simulink model "LTS_testing"  (R2025b)
settings: Solver=ode23t  StartTime=0.0  StopTime=1
model workspace: external: MATLAB File C:\Users\thoma\Documents\ME-Steering-2026\MATLAB\VD\LTS.m (data not in the file)
undefined symbols (not defined in the file): AR26
libraries: vehdynlibtire x4, autolibshared x2, vehdynlibdriver x1, simulink x1, autolibmappedmotor x1, autolibsharedcoupling x1, vehdynlibsteering x1
(part 1 of 2)
settings Model: Creator=thoma  LastModifiedBy=thoma
settings SolverCC: ZeroCrossControl=DisableAll
settings DebuggingCC: UnderSpecifiedDimensionMsg=warning

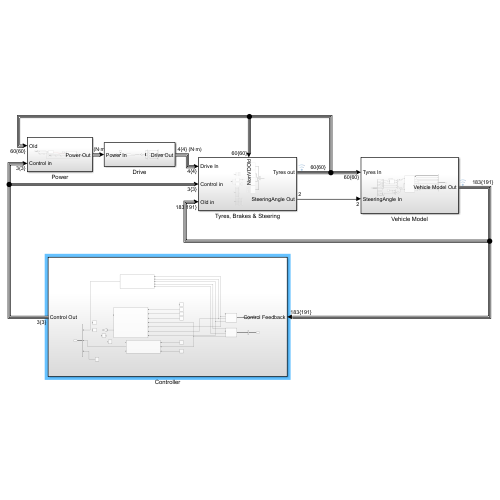
[thumbnail: Simulink's stored preview of the top-level diagram]
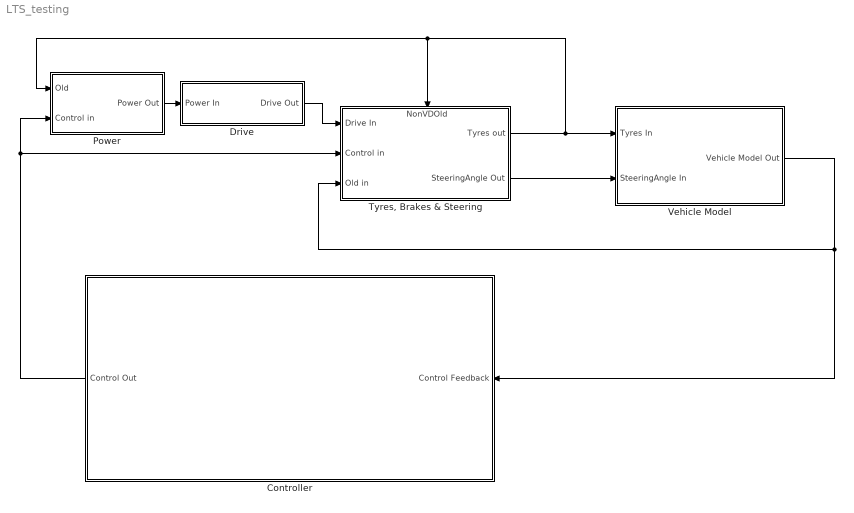
== system LTS_testing ==
  Controller : Subsystem
  Drive : Subsystem
  Power : Subsystem
  "Tyres, Brakes & Steering" : Subsystem
      settings: PortSchema="{\"entries\":[{\"content\":{\"sides\":[{\"content\":{\"connectorIds\":[\"In1\",\"In2\",\"In3\"]},\"type\":\"ConnectorPlacement.EquallySpacedRectSide\",\"uuid\":\"2d0cea8b-83c5-43d0-a9da-df7959890b84\"},{\"content\":{\"connectorIds\":[\"Out1\",\"Out2\"],\"side\":\"RIGHT\"},\"type\":\"ConnectorPlacement.EquallySpacedRectSide\",\"uuid\":\"18a5ce0c-4f74-4e1c-9a31-f96c275e466d\"},{\"content\":{\"connectorIds\":[\"In4\"],\"side\":\"TOP\"},\"type\":\"ConnectorPlacement.EquallySpacedRectSide\",\"uuid\":\"ac68a692-bd3e-4c2d-9cd0-6d8aee15298d\"}]},\"type\":\"ConnectorPlacement.EquallySpacedConnector\",\"uuid\":\"5a266ba3-3c83-4752-af97-895e1d69d679\"}],\"packageUris\":[\"http://schema.mathworks.com/mf0/Connector/R2020b\"],\"version\":\"1.0\"}"
  Vehicle Model : Subsystem
  wires:
  Controller/1(Control Out) -> Power/2(Control in), "Tyres, Brakes & Steering"/2(Control in)
  Drive/1(Drive Out) -> "Tyres, Brakes & Steering"/1(Drive In)
  Power/1(Power Out) -> Drive/1(Power In)
  "Tyres, Brakes & Steering"/1(Tyres out) -> Power/1(Old), "Tyres, Brakes & Steering"/4(NonVDOld), Vehicle Model/1(Tyres In)
  Vehicle Model/1(Vehicle Model Out) -> Controller/1(Control Feedback), "Tyres, Brakes & Steering"/3(Old in)
  "Tyres, Brakes & Steering"/2(SteeringAngle Out) -> Vehicle Model/2(SteeringAngle In)

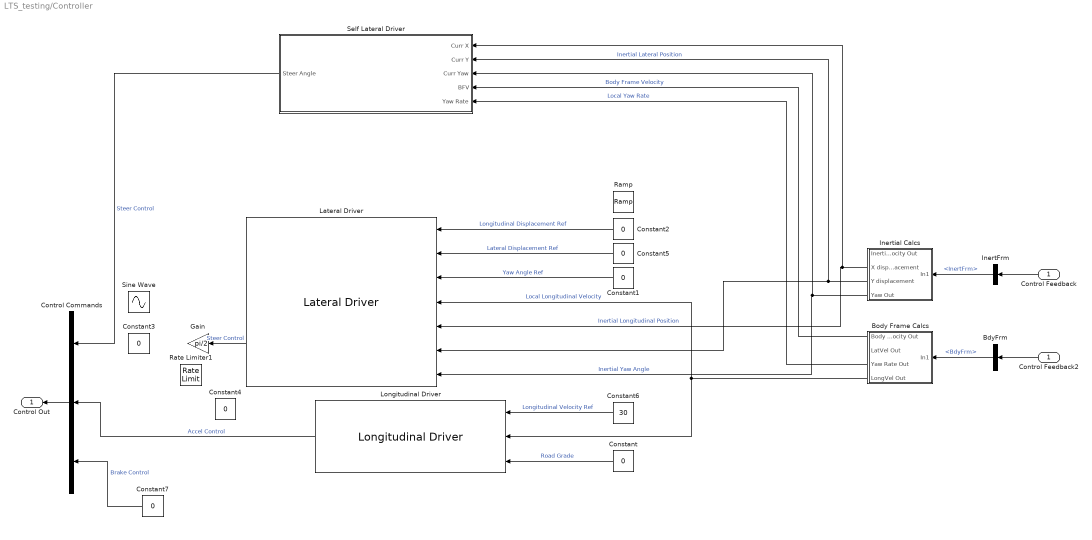
== system LTS_testing/Controller ==
  Control Feedback : Inport
  BdyFrm : BusSelector  OutputSignals=Info.BdyFrm
  Body Frame Calcs : Subsystem
  Constant{,1..5,7} (7 alike) : Constant  Value=0
  Constant6 : Constant  Value=30
  Control Commands : BusCreator  Inputs=3
  Control Feedback2 : InportShadow
  Gain : Gain  Gain=pi/2
  InertFrm : BusSelector  OutputSignals=Info.InertFrm
  Inertial Calcs : Subsystem
  Lateral Driver : vehdynlibdriver/Lateral Driver  extSteerOvr=off  extSteerHld=off  extSteerZero=off  steerOut=off  cntrlTypeLat=Stanley  coordMode=SAE J670 (Z-down)  angUnits=rad  tau=0.1  L=3  vecPose=off  dynamMode=off  PositionGainF=2.5  PositionGainR=2.5  YawRateGain=.2  DelayGain=.2  a=AR26.aLength  b=AR26.bLength  m=AR26.Mass  Cy_f=35000  Cy_r=40000  I=120  Ksteer=18  theta=30*pi/180  aMode=2
  Longitudinal Driver : autolibshared/Longitudinal Driver  extAccelOvr=off  extDecelOvr=off  extAccelHld=off  extDecelHld=off  extAccelZero=off  extDecelZero=off  cntrlType=PI  shftType=None  velUnits=m/s  gearOut=off  Kp=0.7  Ki=0.05  Kff=.1  Kg=0  VehVelVec=[0 100]  KffVec=[.1 .1]  KpVec=[10 10]  KiVec=[5 5]  KgVec=[0 0]  m=1500  Kpt=3000  tau=.1  L=2  aR=200  bR=2.5  cR=.5  g=9.81  vnom=5  Kaw=1  tauerr=.01  tauPt=2  GearInit=0  tShift=.1  pdlVec=[0.1 0.4 0.5 0.9]  upShftTbl=[-1 12.9375 26.4375 39.9375 51.18749999999999 62.4375 72.84375 83.25;-1 16.3125 29.8125 43.3125 54.5624 65.8125 76.78125 87.75;-1 19.6875 33.1875 46.68749999999999 57.9375 69.1875 80.71875 92.25;-1 33 52.5 77.25 100.5 138.75 161.875 185]  dwnShftTbl=[1 9.5625 23.0625 36.5625 47.8125 59.0625 68.90625 78.75;1 12.9375 26.4375 39.9375 51.18749999999999 62.4375 72.84375 83.25;1 16.3125 29.8125 43.3125 54.562499 65.8125 76.78125 87.75;1 19.6875 33.1875 46.68749999999999 57.9375 69.1875 80.71875 92.25]  tClutch=.5  tRev=.5  tPark=120  aMode=2  UpGearVec="[0  1  2  3  4  5  6  7]"  DownGearVec="[1  2  3  4  5  6  7  8]"
      settings: LibrarySourceBlock=vehdynlibdriver/Longitudinal Driver
  Ramp : simulink/Sources/Ramp  slope=35  start=15  InitialOutput=0
  Rate Limiter1 : RateLimiter  RisingSlewLimit=0.5  SampleTimeMode=inherited
  Self Lateral Driver : Subsystem
  Sine Wave : Sin  Amplitude=1.6  Frequency=0.5  SampleTime=0
  Control Out : Outport
  wires:
  Control Commands/1 -> Control Out/1
  Control Feedback/1 -> InertFrm/1
  Control Feedback2/1 -> BdyFrm/1
  Constant/1 -> Longitudinal Driver/3  "Road Grade"
  Constant6/1 -> Longitudinal Driver/1  "Longitudinal Velocity Ref"
  Longitudinal Driver/2 -> Control Commands/2  "Accel Control"
  Constant7/1 -> Control Commands/3  "Brake Control"
  BdyFrm/1 -> Body Frame Calcs/1(In1)  "<BdyFrm>"
  Constant5/1 -> Lateral Driver/2  "Lateral Displacement Ref"
  InertFrm/1 -> Inertial Calcs/1(In1)  "<InertFrm>"
  Inertial Calcs/3(Y displacement) -> Self Lateral Driver/2(Curr Y), Lateral Driver/6  "Inertial Lateral Position"
  Inertial Calcs/4(Yaw Out) -> Self Lateral Driver/3(Curr Yaw), Lateral Driver/7  "Inertial Yaw Angle"
  Body Frame Calcs/4(LongVel Out) -> Longitudinal Driver/2, Lateral Driver/4  "Local Longitudinal Velocity"
  Constant1/1 -> Lateral Driver/3  "Yaw Angle Ref"
  Constant2/1 -> Lateral Driver/1  "Longitudinal Displacement Ref"
  Inertial Calcs/2(X displacement) -> Self Lateral Driver/1(Curr X), Lateral Driver/5  "Inertial Longitudinal Position"
  Lateral Driver/2 -> Gain/1  "Steer Control"
  Body Frame Calcs/1(Body Frame Velocity Out) -> Self Lateral Driver/4(BFV)  "Body Frame Velocity"
  Self Lateral Driver/1(Steer Angle) -> Control Commands/1  "Steer Control"
  Body Frame Calcs/3(Yaw Rate Out) -> Self Lateral Driver/5(Yaw Rate)  "Local Yaw Rate"

== system LTS_testing/Drive ==
  Power In : Inport
  Bus Creator : BusCreator  Inputs=4
  Bus Selector : BusSelector  OutputSignals=Motor Torque (Nm)
  Display : Display
  Gain : Gain
  Gear Ratio : Gain  Gain=AR26.GearRatio
  Multiply{1..4} (4 alike) : Gain
  Drive Out : Outport
  wires:
  Power In/1 -> Bus Selector/1
  Bus Selector/1 -> Gear Ratio/1, Display/1  "<Motor Torque (Nm)>"
  Gear Ratio/1 -> Gain/1
  Multiply4/1 -> Bus Creator/1  "FLDriveTrq"
  Multiply3/1 -> Bus Creator/4  "RRDriveTrq"
  Multiply1/1 -> Bus Creator/2  "FRDriveTrq"
  Multiply2/1 -> Bus Creator/3  "RLDriveTrq"
  Bus Creator/1 -> Drive Out/1
  Gain/1 -> Multiply4/1, Multiply1/1, Multiply3/1, Multiply2/1

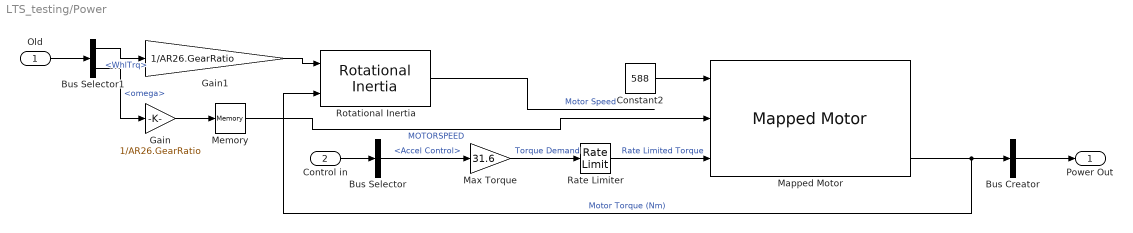
== system LTS_testing/Power ==
  Old : Inport
  Control in : Inport  Port=2
  Bus Creator : BusCreator  Inputs=1
  Bus Selector : BusSelector  OutputSignals=Accel Control
  Bus Selector1 : BusSelector  OutputSignals=FL_Dyn.WhlTrq,FL_Dyn.omega
  Constant2 : Constant  Value=588
  Gain : Gain  Gain=1/AR26.GearRatio
  Gain1 : Gain  Gain=1/AR26.GearRatio
  Mapped Motor : autolibmappedmotor/Mapped Motor  w_Tmax_bp_ext=w_Tmax_bp  Tmax_w_V_ext=Tmax_w_V  w_Tmin_bp_ext=w_Tmin_bp  Tmin_w_V_ext=Tmin_w_V  port_config=Speed  param_by=Maximum torque and power  w_t=[ 0 375 750 800 ]  T_t=[0.09 0.08 0.07 0]  torque_max=31.6  power_max=20000  SpreadsheetTqLimitsFileName=MotorCalibrationImportData.xlsx  Tmax_w_V=[0.09 0.09 0.09;0.08 0.08 0.08;0.07 0.07 0.07;0 0 0]  w_Tmax_bp=[ 0 375 750 800 ]  V_Tmax_bp=[500 750 900]  Tmin_w_V=[-0.09 -0.09 -0.09;-0.08 -0.08 -0.08;-0.07 -0.07 -0.07;0 0 0]  w_Tmin_bp=[ 0 375 750 800 ]  V_Tmin_bp=[500 750 900]  Tc=0.02  param_loss=Single efficiency measurement  SpreadsheetLossFileName=MotorCalibrationImportData.xlsx  SpreadsheetEffFileName=MotorCalibrationImportData.xlsx  eff=95  w_eff=375  T_eff=0.08  Piron=0  Pbase=0  w_eff_bp=[-8000 -4000 0 4000 8000]  T_eff_bp=[0 0.03 0.06 0.09]  Temp_eff_bp=[233.15 293.15 373.15]  V_eff_bp=[500 700 900]  losses_table=[1.49 1.67 2.21 3.10; 0.42 0.69 1.14 2.03; 0.06 0.24 0.78 1.68; 0.42 0.69 1.14 2.03; 1.49 1.67 2.21 3.10]  losses_table_3d=cat(3,1.05*[1.49 1.67 2.21 3.10; 0.42 0.69 1.14 2.03; 0.06 0.24 0.78 1.68; 0.42 0.69 1.14 2.03; 1.49 1.67 2.21 3.10],[1.49 1.67 2.21 3.10; 0.42 0.69 1.14 2.03; 0.06 0.24 0.78 1.68; 0.42 0.69 1.14 2.03; 1.49 1.67 2.21 3.10],1.03*[1.49 1.67 2.21 3.10; 0.42 0.69 1.14 2.03; 0.06 0.24 0.78 1.68; 0.42 0.69 1.14 2.03; 1.49 1.67 2.21 3.10])  losses_table_4d=cat(4,cat(3,[1.5645 0.441 0.063 0.441 1.5645;1.7535 0.7245 0.252 0.7245 1.7535;2.3205 1.197 0.819 1.197 2.3205;3.255 2.1315 1.764 2.1315 3.255],[1.5645 0.441 0.063 0.441 1.5645;1.7535 0.7245 0.252 0.7245 1.7535;2.3205 1.197 0.819 1.197 2.3205;3.255 2.1315 1.764 2.1315 3.255],[1.5645 0.441 0.063 0.441 1.5645;1.7535 0.7245 0.252 0.7245 1.7535;2.3205 1.197 0.819 1.197 2.3205;3.255 2.1315 1.764 2.1315 3.255]),cat(3,[1.49 0.42 0.06 0.42 1.49;1.67 0.69 0.24 0.69 1.67;2.21 1.14 0.78 1.14 2.21;3.1 2.03 1.68 2.03 3.1],[1.49 0.42 0.06 0.42 1.49;1.67 0.69 0.24 0.69 1.67;2.21 1.14 0.78 1.14 2.21;3.1 2.03 1.68 2.03 3.1],[1.49 0.42 0.06 0.42 1.49;1.67 0.69 0.24 0.69 1.67;2.21 1.14 0.78 1.14 2.21;3.1 2.03 1.68 2.03 3.1]),cat(3,[1.5347 0.4326 0.0618 0.4326 1.5347;1.7201 0.7107 0.2472 0.7107 1.7201;2.2763 1.1742 0.8034 1.1742 2.2763;3.193 2.0909 1.7304 2.0909 3.193],[1.5347 0.4326 0.0618 0.4326 1.5347;1.7201 0.7107 0.2472 0.7107 1.7201;2.2763 1.1742 0.8034 1.1742 2.2763;3.193 2.0909 1.7304 2.0909 3.193],[1.5347 0.4326 0.0618 0.4326 1.5347;1.7201 0.7107 0.2472 0.7107 1.7201;2.2763 1.1742 0.8034 1.1742 2.2763;3.193 2.0909 1.7304 2.0909 3.193]))  efficiency_table=[95 95 95 95; 95 95 95 95; 95 95 95 95; 95 95 95 95; 95 95 95 95]  efficiency_table_3d=cat(3,90*ones(5,4),95*ones(5,4),92*ones(5,4))  efficiency_table_4d=cat(4,cat(3,90*ones(5,4)',90*ones(5,4)',90*ones(5,4)'),cat(3,95*ones(5,4)',95*ones(5,4)',95*ones(5,4)'),cat(3,92*ones(5,4)',92*ones(5,4)',92*ones(5,4)'))  J=5e-6  b=1e-5  omega_o=0  T_t_extended=[0 0.07 0.08 0.09 0.08 0.07 0]  w_t_extended=[-800 -750 -375 0 375 750 800]  KLossIron=0  KLossCopper=0  x_w_eff_vec=[-8000 -4000 0 4000 8000]  x_T_eff_vec=[-0.09 -0.06 -0.03 0 0.03 0.06 0.09]  x_tmp_eff_vec=[233.15 293.15 373.15]  x_V_eff_vec=[500 700 900]  x_losses_mat=[3.1 2.21 1.67 1.49 1.67 2.21 3.1;2.03 1.14 0.69 0.42 0.69 1.14 2.03;1.68 0.78 0.24 0.06 0.24 0.78 1.68;2.03 1.14 0.69 0.42 0.69 1.14 2.03;3.1 2.21 1.67 1.49 1.67 2.21 3.1]  x_losses_mat_3d=cat(3,[3.255 2.3205 1.7535 1.5645 1.7535 2.3205 3.255;2.1315 1.197 0.7245 0.441 0.7245 1.197 2.1315;1.764 0.819 0.252 0.063 0.252 0.819 1.764;2.1315 1.197 0.7245 0.441 0.7245 1.197 2.1315;3.255 2.3205 1.7535 1.5645 1.7535 2.3205 3.255],[3.1 2.21 1.67 1.49 1.67 2.21 3.1;2.03 1.14 0.69 0.42 0.69 1.14 2.03;1.68 0.78 0.24 0.06 0.24 0.78 1.68;2.03 1.14 0.69 0.42 0.69 1.14 2.03;3.1 2.21 1.67 1.49 1.67 2.21 3.1],[3.193 2.2763 1.7201 1.5347 1.7201 2.2763 3.193;2.0909 1.1742 0.7107 0.4326 0.7107 1.1742 2.0909;1.7304 0.8034 0.2472 0.0618 0.2472 0.8034 1.7304;2.0909 1.1742 0.7107 0.4326 0.7107 1.1742 2.0909;3.193 2.2763 1.7201 1.5347 1.7201 2.2763 3.193])  x_losses_mat_4d=cat(4,cat(3,[1.5645 0.441 0.063 0.441 1.5645;1.7535 0.7245 0.252 0.7245 1.7535;2.3205 1.197 0.819 1.197 2.3205;3.255 2.1315 1.764 2.1315 3.255],[1.5645 0.441 0.063 0.441 1.5645;1.7535 0.7245 0.252 0.7245 1.7535;2.3205 1.197 0.819 1.197 2.3205;3.255 2.1315 1.764 2.1315 3.255],[1.5645 0.441 0.063 0.441 1.5645;1.7535 0.7245 0.252 0.7245 1.7535;2.3205 1.197 0.819 1.197 2.3205;3.255 2.1315 1.764 2.1315 3.255]),cat(3,[1.49 0.42 0.06 0.42 1.49;1.67 0.69 0.24 0.69 1.67;2.21 1.14 0.78 1.14 2.21;3.1 2.03 1.68 2.03 3.1],[1.49 0.42 0.06 0.42 1.49;1.67 0.69 0.24 0.69 1.67;2.21 1.14 0.78 1.14 2.21;3.1 2.03 1.68 2.03 3.1],[1.49 0.42 0.06 0.42 1.49;1.67 0.69 0.24 0.69 1.67;2.21 1.14 0.78 1.14 2.21;3.1 2.03 1.68 2.03 3.1]),cat(3,[1.5347 0.4326 0.0618 0.4326 1.5347;1.7201 0.7107 0.2472 0.7107 1.7201;2.2763 1.1742 0.8034 1.1742 2.2763;3.193 2.0909 1.7304 2.0909 3.193],[1.5347 0.4326 0.0618 0.4326 1.5347;1.7201 0.7107 0.2472 0.7107 1.7201;2.2763 1.1742 0.8034 1.1742 2.2763;3.193 2.0909 1.7304 2.0909 3.193],[1.5347 0.4326 0.0618 0.4326 1.5347;1.7201 0.7107 0.2472 0.7107 1.7201;2.2763 1.1742 0.8034 1.1742 2.2763;3.193 2.0909 1.7304 2.0909 3.193]))  CalLossMapData={}  CalLossWithTempMapData={}  aMode=2  RefBlkName='autolibmappedmotor/Mapped Motor'
      settings: LibrarySourceBlock=vdynlib/Powertrain/Propulsion/Mapped Motor
  Max Torque : Gain  Gain=31.6
  Memory : Memory
  Rate Limiter : RateLimiter  RisingSlewLimit=0.1  FallingSlewLimit=-100  SampleTimeMode=inherited
  Rotational Inertia : autolibsharedcoupling/Rotational Inertia  port_config=Simulink  extInfo=off  externJ=off  J=.01  b=.001  omega_o=0  blkID=0  aMode=2
      settings: LibrarySourceBlock=vdynlib/Powertrain/Drivetrain/Couplings/Rotational Inertia
  Power Out : Outport
  wires:
  Constant2/1 -> Mapped Motor/1
  Old/1 -> Bus Selector1/1
  Mapped Motor/3 -> Rotational Inertia/2, Bus Creator/1  "Motor Torque (Nm)"
  Bus Creator/1 -> Power Out/1
  Control in/1 -> Bus Selector/1
  Bus Selector/1 -> Max Torque/1  "<Accel Control>"
  Max Torque/1 -> Rate Limiter/1  "Torque Demand"
  Rotational Inertia/1 -> ?  "Motor Speed"
  Bus Selector1/1 -> Gain1/1  "<WhlTrq>"
  Gain1/1 -> Rotational Inertia/1
  Rate Limiter/1 -> Mapped Motor/3  "Rate Limited Torque"
  Bus Selector1/2 -> Gain/1  "<omega>"
  Gain/1 -> Memory/1
  Memory/1 -> Mapped Motor/2  "MOTORSPEED"

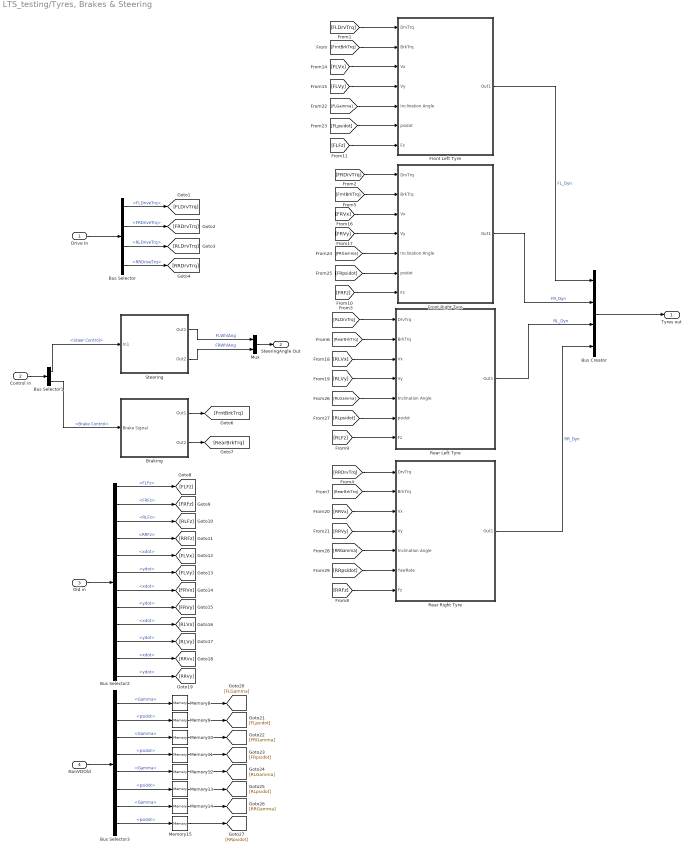
== system LTS_testing/Tyres, Brakes & Steering ==
  Drive In : Inport
  Control in : Inport  Port=2
  Old in : Inport  Port=3
  NonVDOld : Inport  Port=4
  Braking : Subsystem
  Bus Creator : BusCreator  Inputs=4
  Bus Selector : BusSelector  OutputSignals=FLDriveTrq,FRDriveTrq,RLDriveTrq,RRDriveTrq
  Bus Selector1 : BusSelector  OutputSignals=Steer Control,Brake Control
  Bus Selector2 : BusSelector  OutputSignals=FLFz,FRFz,RLFz,RRFz,Info.BdyFrm.FrntAxl.Lft.Vel.xdot,Info.BdyFrm.FrntAxl.Lft.Vel.ydot,Info.BdyFrm.FrntAxl.Rght.Vel.xdot,Info.BdyFrm.FrntAxl.Rght.Vel.ydot,Info.BdyFrm.RearAxl.Lft.Vel.xdot,Info.BdyFrm.RearAxl.Lft.Vel.ydot,Info.BdyFrm.RearAxl.Rght.Vel.xdot,Info.BdyFrm.RearAxl.Rght.Vel.ydot
  Bus Selector3 : BusSelector  OutputSignals=FL_Dyn.Gamma,FL_Dyn.psidot,FR_Dyn.Gamma,FR_Dyn.psidot,RL_Dyn.Gamma,RL_Dyn.psidot,RR_Dyn.Gamma,RR_Dyn.psidot
  Front Left Tyre : Subsystem
  Front Right Tyre : Subsystem
  Memory{8..15} (8 alike) : Memory
  Mux : Mux  Inputs=2
  Rear Left Tyre : Subsystem
  Rear Right Tyre : Subsystem
  Steering : Subsystem
  Tyres out : Outport
  SteeringAngle Out : Outport  Port=2
  wires:
  Bus Creator/1 -> Tyres out/1
  Front Left Tyre/1(Out1) -> Bus Creator/1  "FL_Dyn"
  Front Right Tyre/1(Out1) -> Bus Creator/2  "FR_Dyn"
  Rear Left Tyre/1(Out1) -> Bus Creator/3  "RL_Dyn"
  Rear Right Tyre/1(Out1) -> Bus Creator/4  "RR_Dyn"
  Control in/1 -> Bus Selector1/1
  Bus Selector1/1 -> Steering/1(In1)  "<Steer Control>"
  Steering/1(Out1) -> Mux/1  "FLWhlAng"
  Steering/2(Out2) -> Mux/2  "FRWhlAng"
  Braking/1(Out1) -> [FrntBrkTrq]
  Braking/2(Out2) -> [RearBrkTrq]
  Bus Selector/1 -> [FLDrvTrq]  "<FLDriveTrq>"
  Drive In/1 -> Bus Selector/1
  Bus Selector/4 -> [RRDrvTrq]  "<RRDriveTrq>"
  Bus Selector/3 -> [RLDrvTrq]  "<RLDriveTrq>"
  Bus Selector/2 -> [FRDrvTrq]  "<FRDriveTrq>"
  [FLDrvTrq] -> Front Left Tyre/1(DrvTrq)
  [FrntBrkTrq] -> Front Left Tyre/2(BrkTrq)
  [FRDrvTrq] -> Front Right Tyre/1(DrvTrq)
  [FrntBrkTrq] -> Front Right Tyre/2(BrkTrq)
  [RLDrvTrq] -> Rear Left Tyre/1(DrvTrq)
  [RearBrkTrq] -> Rear Left Tyre/2(BrkTrq)
  [RRDrvTrq] -> Rear Right Tyre/1(DrvTrq)
  [RearBrkTrq] -> Rear Right Tyre/2(BrkTrq)
  Bus Selector1/2 -> Braking/1(Brake Signal)  "<Brake Control>"
  [FRFz] -> Front Right Tyre/7(Fz)
  [RLFz] -> Rear Left Tyre/7(Fz)
  [RRFz] -> Rear Right Tyre/7(Fz)
  Old in/1 -> Bus Selector2/1
  [FLFz] -> Front Left Tyre/7(Fz)
  [FRGamma] -> Front Right Tyre/5(Inclination Angle)
  [FLGamma] -> Front Left Tyre/5(Inclination Angle)
  [RLGamma] -> Rear Left Tyre/5(Inclination Angle)
  [RRGamma] -> Rear Right Tyre/5(Inclination Angle)
  [RLVx] -> Rear Left Tyre/3(Vx)
  [RLVy] -> Rear Left Tyre/4(Vy)
  [RRVx] -> Rear Right Tyre/3(Vx)
  [RRVy] -> Rear Right Tyre/4(Vy)
  [FLVy] -> Front Left Tyre/4(Vy)
  [FLVx] -> Front Left Tyre/3(Vx)
  [FRVy] -> Front Right Tyre/4(Vy)
  [FRVx] -> Front Right Tyre/3(Vx)
  NonVDOld/1 -> Bus Selector3/1
  Bus Selector3/1 -> Memory8/1  "<Gamma>"
  Bus Selector3/2 -> Memory9/1  "<psidot>"
  Bus Selector3/3 -> Memory10/1  "<Gamma>"
  Bus Selector3/4 -> Memory11/1  "<psidot>"
  Bus Selector3/5 -> Memory12/1  "<Gamma>"
  Bus Selector3/6 -> Memory13/1  "<psidot>"
  Bus Selector3/7 -> Memory14/1  "<Gamma>"
  Bus Selector3/8 -> Memory15/1  "<psidot>"
  Memory8/1 -> [FLGamma]
  Memory9/1 -> [FLpsidot]
  [FLpsidot] -> Front Left Tyre/6(psidot)
  [FRpsidot] -> Front Right Tyre/6(psidot)
  [RLpsidot] -> Rear Left Tyre/6(psidot)
  [RRpsidot] -> Rear Right Tyre/6(YawRate)
  Memory10/1 -> [FRGamma]
  Memory11/1 -> [FRpsidot]
  Memory12/1 -> [RLGamma]
  Memory13/1 -> [RLpsidot]
  Memory14/1 -> [RRGamma]
  Memory15/1 -> [RRpsidot]
  Bus Selector2/2 -> [FRFz]  "<FRFz>"
  Bus Selector2/3 -> [RLFz]  "<RLFz>"
  Bus Selector2/5 -> [FLVx]  "<xdot>"
  Bus Selector2/6 -> [FLVy]  "<ydot>"
  Bus Selector2/7 -> [FRVx]  "<xdot>"
  Bus Selector2/8 -> [FRVy]  "<ydot>"
  Bus Selector2/9 -> [RLVx]  "<xdot>"
  Bus Selector2/10 -> [RLVy]  "<ydot>"
  Bus Selector2/11 -> [RRVx]  "<xdot>"
  Bus Selector2/12 -> [RRVy]  "<ydot>"
  Bus Selector2/1 -> [FLFz]  "<FLFz>"
  Bus Selector2/4 -> [RRFz]  "<RRFz>"
  Mux/1 -> SteeringAngle Out/1

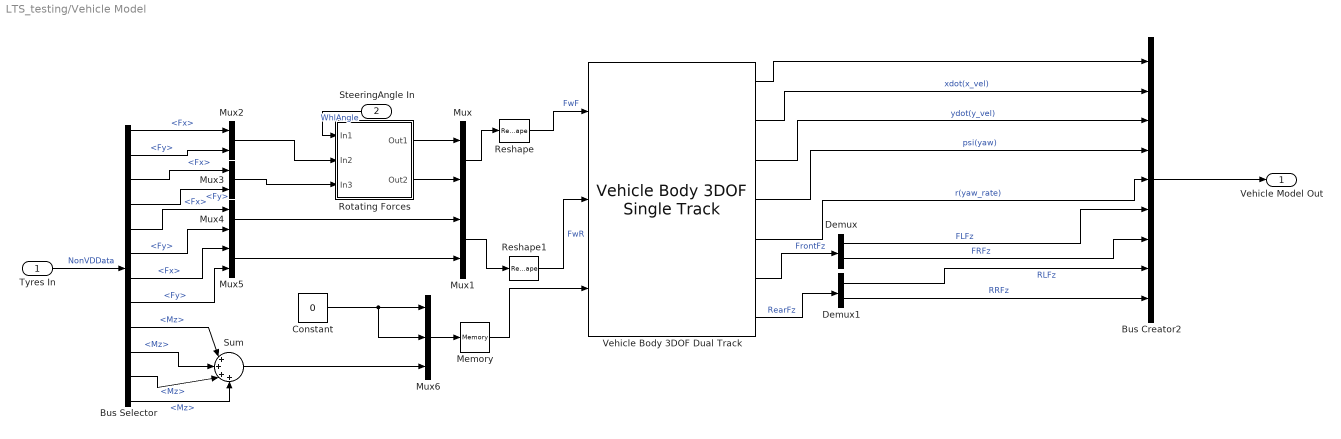
== system LTS_testing/Vehicle Model ==
  Tyres In : Inport
  SteeringAngle In : Inport  Port=2
  Bus Creator2 : BusCreator  Inputs=9
  Bus Selector : BusSelector  OutputSignals=FL_Dyn.Fx,FL_Dyn.Fy,FR_Dyn.Fx,FR_Dyn.Fy,RL_Dyn.Fx,RL_Dyn.Fy,RR_Dyn.Fx,RR_Dyn.Fy,FL_Dyn.Mz,FR_Dyn.Mz,RL_Dyn.Mz,RR_Dyn.Mz
  Constant : Constant  Value=0
  Demux : Demux  Outputs=2
  Demux1 : Demux  Outputs=2
  Memory : Memory
  Mux{,1..5} (6 alike) : Mux  Inputs=2
  Mux6 : Mux  Inputs=3
  Reshape : Reshape  OutputDimensionality=Customize  OutputDimensions=[2,2]
  Reshape1 : Reshape  OutputDimensionality=Customize  OutputDimensions=[2,2]
  Rotating Forces : Subsystem
  Sum : Sum  Inputs=|++++
  Vehicle Body 3DOF Dual Track : autolibshared/Vehicle Body 3DOF Single Track  trackMode=Dual  inputMode=External forces  frontSteerMode=off  rearSteerMode=off  windMode=off  muMode=off  extFMode=off  extMMode=on  htchFMode=off  htchMMode=off  extXo=off  extpsio=off  extxdoto=off  extro=off  extYo=off  extTamb=off  extydoto=off  aMode=2  NF=2  NR=2  m=AR26.Mass  a=AR26.aLength  b=AR26.bLength  h=AR26.CGHeight  dh=1  hh=0.2  X_o=0  xdot_o=AR26.Vx0  CalphaMode=off  sigmaMode=on  d=AR26.CGLateral  hl=0  w=[AR26.FrontTrackwidth,AR26.RearTrackWidth]  Cy_f=12e3  Cy_r=11e3  sigma_f=.1  sigma_r=.1  alpha_f_brk=[-0.785, -0.628, -0.471, -0.314, -0.157, 0.000, 0.157, 0.314, 0.471, 0.628, 0.785]  Cy_f_data=[2000, 3000, 4000, 5500, 7000, 9000, 7000, 5500, 4000, 3000, 2000]  alpha_r_brk=[-0.785, -0.628, -0.471, -0.314, -0.157, 0.000, 0.157, 0.314, 0.471, 0.628, 0.785]  Cy_r_data=[2000, 3000, 4000, 5500, 7000, 9000, 7000, 5500, 4000, 3000, 2000]  Y_o=0  ydot_o=0  Izz=AR26.Izz  psi_o=0  r_o=0  Af=0.81  Cd=1.4  Cl=4.230  Cpm=.1  beta_w=[0 0.01:0.01:0.3]  Cs=[0:0.03:0.9]  Cym=[0 1e-6:0.01:0.3]  Pabs=101325  Tair=273  g=9.81  mu=1  xdot_tol=.01  Fznom=5000  Fxtire_sat=7e4  Fytire_sat=7e4  longOff=0  latOff=0  vertOff=0  wrapAng=off
      settings: LibrarySourceBlock=vehdynlibeom/Vehicle Body 3DOF Dual Track
  Vehicle Model Out : Outport
  wires:
  Tyres In/1 -> Bus Selector/1  "NonVDData"
  Bus Selector/3 -> Mux3/1  "<Fx>"
  Bus Selector/5 -> Mux4/1  "<Fx>"
  Bus Selector/7 -> Mux5/1  "<Fx>"
  Vehicle Body 3DOF Dual Track/2 -> Bus Creator2/2  "xdot(x_vel)"
  Vehicle Body 3DOF Dual Track/7 -> Demux1/1  "RearFz"
  Vehicle Body 3DOF Dual Track/3 -> Bus Creator2/3  "ydot(y_vel)"
  Vehicle Body 3DOF Dual Track/4 -> Bus Creator2/4  "psi(yaw)"
  Vehicle Body 3DOF Dual Track/5 -> Bus Creator2/5  "r(yaw_rate)"
  Vehicle Body 3DOF Dual Track/6 -> Demux/1  "FrontFz"
  Demux/1 -> Bus Creator2/6  "FLFz"
  Demux/2 -> Bus Creator2/7  "FRFz"
  Demux1/1 -> Bus Creator2/8  "RLFz"
  Demux1/2 -> Bus Creator2/9  "RRFz"
  Bus Selector/1 -> Mux2/1  "<Fx>"
  Bus Selector/2 -> Mux2/2  "<Fy>"
  Bus Selector/4 -> Mux3/2  "<Fy>"
  Bus Selector/6 -> Mux4/2  "<Fy>"
  Bus Selector/8 -> Mux5/2  "<Fy>"
  Mux/1 -> Reshape/1
  Mux1/1 -> Reshape1/1
  Bus Creator2/1 -> Vehicle Model Out/1
  Vehicle Body 3DOF Dual Track/1 -> Bus Creator2/1
  Mux2/1 -> Rotating Forces/2(In2)
  Mux3/1 -> Rotating Forces/3(In3)
  Mux4/1 -> Mux1/1
  Mux5/1 -> Mux1/2
  SteeringAngle In/1 -> Rotating Forces/1(In1)  "WhlAngle"
  Reshape1/1 -> Vehicle Body 3DOF Dual Track/2  "FwR"
  Reshape/1 -> Vehicle Body 3DOF Dual Track/1  "FwF"
  Rotating Forces/1(Out1) -> Mux/1
  Rotating Forces/2(Out2) -> Mux/2
  Bus Selector/9 -> Sum/1  "<Mz>"
  Bus Selector/10 -> Sum/2  "<Mz>"
  Bus Selector/11 -> Sum/3  "<Mz>"
  Bus Selector/12 -> Sum/4  "<Mz>"
  Sum/1 -> Mux6/3
  Constant/1 -> Mux6/2, Mux6/1
  Mux6/1 -> Memory/1
  Memory/1 -> Vehicle Body 3DOF Dual Track/3

== system LTS_testing/Controller/Body Frame Calcs ==
  In1 : Inport
  Bus Selector : BusSelector  OutputSignals=Cg.Vel.xdot,Cg.Vel.ydot,FrntAxl.Steer.WhlAngFL,FrntAxl.Steer.WhlAngFR,Cg.Ang.Beta,Cg.AngVel.r,Cg.DCM
  Integrator : Integrator
  Integrator1 : Integrator
  Velocity : Math  Operator=hypot
  Body Frame Velocity Out : Outport
  LatVel Out : Outport  Port=2
  Yaw Rate Out : Outport  Port=3
  LongVel Out : Outport  Port=4
  wires:
  In1/1 -> Bus Selector/1
  Bus Selector/2 -> Velocity/2, Integrator1/1, LatVel Out/1  "<ydot>"
  Bus Selector/1 -> LongVel Out/1, Integrator/1, Velocity/1  "<xdot>"
  Velocity/1 -> Body Frame Velocity Out/1  "Body Frame Velocity"
  Bus Selector/6 -> Yaw Rate Out/1  "<r>"

== system LTS_testing/Controller/Inertial Calcs ==
  In1 : Inport
  Bus Selector : BusSelector  OutputSignals=Cg.Vel.Xdot,Cg.Vel.Ydot,Cg.Ang.psi,Cg.Disp.X,Cg.Disp.Y
  Hypot : Math  Operator=hypot
  Inertial Velocity Out : Outport
  X displacement : Outport  Port=2
  Y displacement : Outport  Port=3
  Yaw Out : Outport  Port=4
  wires:
  In1/1 -> Bus Selector/1
  Bus Selector/2 -> Hypot/2  "<Ydot>"
  Bus Selector/1 -> Hypot/1  "<Xdot>"
  Hypot/1 -> Inertial Velocity Out/1
  Bus Selector/3 -> Yaw Out/1  "<psi>"
  Bus Selector/4 -> X displacement/1  "<X>"
  Bus Selector/5 -> Y displacement/1  "<Y>"

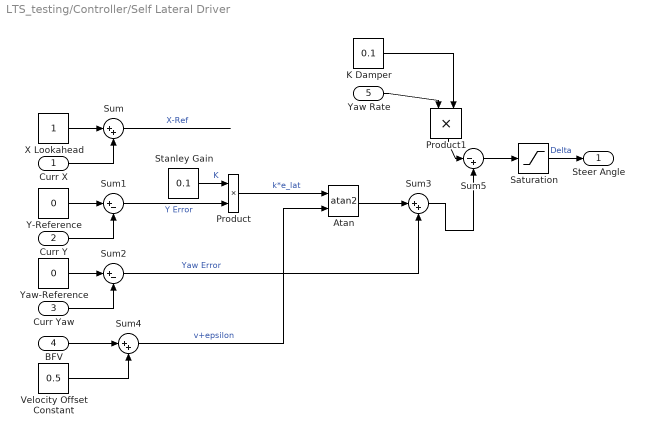
== system LTS_testing/Controller/Self Lateral Driver ==
  Curr X : Inport
  Curr Y : Inport  Port=2
  Curr Yaw : Inport  Port=3
  BFV : Inport  Port=4
  Yaw Rate : Inport  Port=5
  Atan : Trigonometry  Operator=atan2
  K Damper : Constant  Value=0.1
  Product : Product
  Product1 : Product
  Saturation : Saturate  UpperLimit=1.6  LowerLimit=-1.6
  Stanley Gain : Constant  Value=0.1
  Sum : Sum  Inputs=|++
  Sum1 : Sum  Inputs=|+-
  Sum2 : Sum  Inputs=|+-
  Sum3 : Sum  Inputs=|++
  Sum4 : Sum  Inputs=|++
  Sum5 : Sum  Inputs=|-+
  Velocity Offset Constant : Constant  Value=0.5
  X Lookahead : Constant
  Y-Reference : Constant  Value=0
  Yaw-Reference : Constant  Value=0
  Steer Angle : Outport
  wires:
  Curr Y/1 -> Sum1/2
  Curr Yaw/1 -> Sum2/2
  Sum1/1 -> Product/2  "Y Error"
  Curr X/1 -> Sum/2
  X Lookahead/1 -> Sum/1
  Sum/1 -> ?  "X-Ref"
  Y-Reference/1 -> Sum1/1
  Yaw-Reference/1 -> Sum2/1
  Sum2/1 -> Sum3/2  "Yaw Error"
  Saturation/1 -> Steer Angle/1  "Delta"
  Atan/1 -> Sum3/1
  Stanley Gain/1 -> Product/1  "K"
  BFV/1 -> Sum4/1
  Velocity Offset Constant/1 -> Sum4/2
  Sum4/1 -> Atan/2  "v+epsilon"
  Product/1 -> Atan/1  "k*e_lat"
  Sum3/1 -> Sum5/2
  K Damper/1 -> Product1/2
  Yaw Rate/1 -> Product1/1
  Product1/1 -> Sum5/1
  Sum5/1 -> Saturation/1

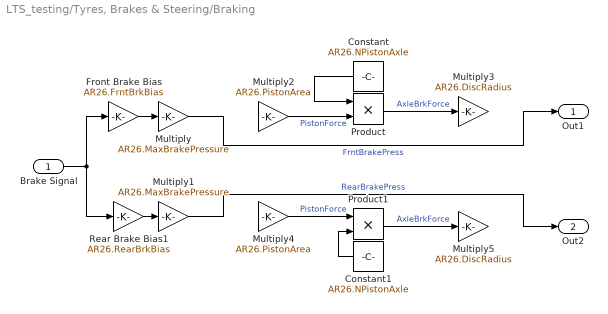
== system LTS_testing/Tyres, Brakes & Steering/Braking ==
  Brake Signal : Inport
  Constant : Constant  Value=AR26.NPistonAxle
  Constant1 : Constant  Value=AR26.NPistonAxle
  Front Brake Bias : Gain  Gain=AR26.FrntBrkBias
  Multiply : Gain  Gain=AR26.MaxBrakePressure
  Multiply1 : Gain  Gain=AR26.MaxBrakePressure
  Multiply2 : Gain  Gain=AR26.PistonArea
  Multiply3 : Gain  Gain=AR26.DiscRadius
  Multiply4 : Gain  Gain=AR26.PistonArea
  Multiply5 : Gain  Gain=AR26.DiscRadius
  Product : Product
  Product1 : Product
  Rear Brake Bias1 : Gain  Gain=AR26.RearBrkBias
  Out1 : Outport
  Out2 : Outport  Port=2
  wires:
  Brake Signal/1 -> Front Brake Bias/1, Rear Brake Bias1/1
  Front Brake Bias/1 -> Multiply/1
  Rear Brake Bias1/1 -> Multiply1/1
  Multiply/1 -> Out1/1  "FrntBrakePress"
  Multiply1/1 -> Out2/1  "RearBrakePress"
  Constant/1 -> Product/1
  Multiply2/1 -> Product/2  "PistonForce"
  Product/1 -> Multiply3/1  "AxleBrkForce"
  Multiply4/1 -> Product1/1  "PistonForce"
  Constant1/1 -> Product1/2
  Product1/1 -> Multiply5/1  "AxleBrkForce"

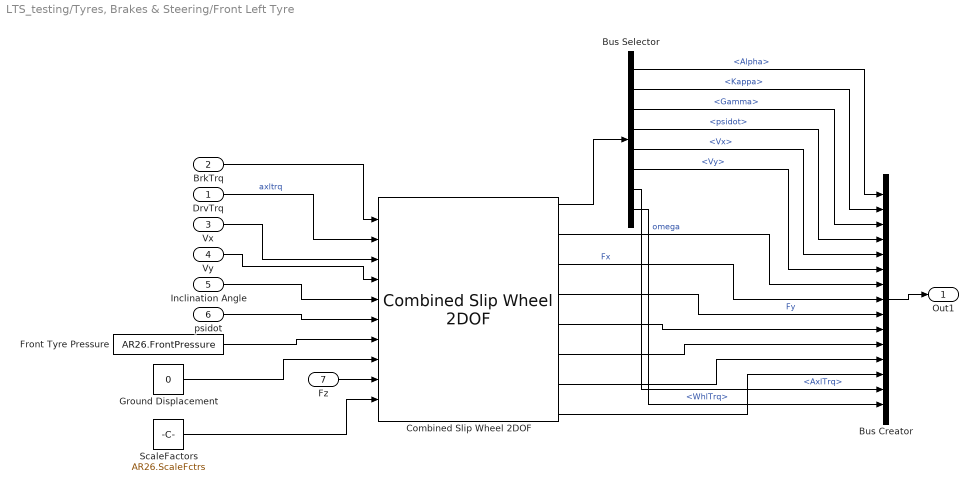
== system LTS_testing/Tyres, Brakes & Steering/Front Left Tyre ==
  DrvTrq : Inport
  BrkTrq : Inport  Port=2
  Vx : Inport  Port=3
  Vy : Inport  Port=4
  Inclination Angle : Inport  Port=5
  psidot : Inport  Port=6
  Fz : Inport  Port=7
  Bus Creator : BusCreator  Inputs=15
  Bus Selector : BusSelector  OutputSignals=Alpha,Kappa,Gamma,psidot,Vx,Vy,AxlTrq,WhlTrq
  Combined Slip Wheel 2DOF : vehdynlibtire/Combined Slip Wheel 2DOF  tireType=External file  tireParamSet=C:\Users\thoma\Documents\ME-Steering-2026\MATLAB\VD\left.tir  vertType=Magic Formula  plySteer=off  turnslip=off  BrakeType=Disc  mu_static=.3  mu_kinetic=.2  drum_abore=0.0508  drum_a=0.123  drum_c=0.212  drum_r=0.15  drum_theta1=0  drum_theta2=126  disk_abore=AR26.PistonDiam  Rm=AR26.DiscRadius  num_pads=4  brake_p_bpt=[1 11.4736842105263 21.9473684210526 32.4210526315789 42.8947368421053 53.3684210526316 63.8421052631579 74.3157894736842 84.7894736842105 95.2631578947368 105.736842105263 116.210526315789 126.684210526316 137.157894736842 147.631578947368 158.105263157895 168.578947368421 179.052631578947 189.526315789474 200]  brake_n_bpt=[0 52.6315789473684 105.263157894737 157.894736842105 210.526315789474 263.157894736842 315.789473684211 368.421052631579 421.052631578947 473.684210526316 526.315789473684 578.947368421053 631.578947368421 684.210526315789 736.842105263158 789.473684210526 842.105263157895 894.736842105263 947.368421052632 1000]  f_brake_t=[43.4900602404453 42.5056030554862 41.5350898940194 40.5780454442085 39.6340111501808 38.7025443887544 37.7832176914519 36.8756180088306 35.9793460143796 35.0940154454303 34.2192524787115 33.3546951383474 32.4999927342521 31.6548053290159 30.8188032315107 29.991666515561 29.1730845621415 28.362755623661 27.5603864089927 26.765691687993;498.991217495636 487.695866636631 476.560505099801 465.579679307235 454.748127933653 444.060772460445 433.51270824929 423.099196101319 412.81565427025 402.657650900201 392.620896861006 382.701238955775 372.894653477208 363.197240090814 353.605216024701 344.114910546964 334.722759712992 325.425301366216 316.219170376863 307.10109410434;954.492374750826 932.886130217776 911.585920305583 890.581313170261 869.862244717126 849.419000532136 829.242198807128 809.322774193808 789.651962526121 770.221286354971 751.0225412433 732.047782773203 713.289314220164 694.739674852612 676.391628817892 658.238154578366 640.272434863842 622.48784710877 604.877954344734 587.436496520688;1409.99353200602 1378.07639379892 1346.61133551136 1315.58294703329 1284.9763615006 1254.77722860383 1224.97168936497 1195.5463522863 1166.48827078199 1137.78492180974 1109.42418562559 1081.39432659063 1053.68397496312 1026.28210961441 999.178041611083 972.361398609768 945.822110014692 919.550392851325 893.536738312604 867.771898937035;1865.49468926121 1823.26665738007 1781.63675071715 1740.58458089631 1700.09047828407 1660.13545667552 1620.7011799228 1581.76993037878 1543.32457903786 1505.34855726451 1467.82583000789 1430.74087040806 1394.07863570608 1357.82454437621 1321.96445440427 1286.48464264117 1251.37178516554 1216.61293859388 1182.19552228048 1148.10730135338;2320.9958465164 2268.45692096121 2216.66216592293 2165.58621475934 2115.20459506754 2065.49368474721 2016.43067048064 1967.99350847127 1920.16088729373 1872.91219271928 1826.22747439018 1780.08741422549 1734.47329644903 1689.36697913801 1644.75086719747 1600.60788667257 1556.92146031639 1513.67548433643 1470.85430624835 1428.44270376973;2776.49700377159 2713.64718454235 2651.68758112871 2590.58784862237 2530.31871185102 2470.8519128189 2412.16016103848 2354.21708656376 2296.9971955496 2240.47582817405 2184.62911877248 2129.43395804292 2074.86795719199 2020.9094138998 1967.53727999066 1914.73113070398 1862.47113546724 1810.73803007899 1759.51309021622 1708.77810618608;3231.99816102678 3158.8374481235 3086.71299633449 3015.58948248539 2945.43282863449 2876.21014089059 2807.88965159632 2740.44066465625 2673.83350380547 2608.03946362882 2543.03076315477 2478.78050186034 2415.26261793494 2352.4518486616 2290.32369278385 2228.85437473538 2168.02081061809 2107.80057582154 2048.17187418409 1989.11350860242;3687.49931828197 3604.02771170464 3521.73841154027 3440.59111634842 3360.54694541796 3281.56836896228 3203.61914215416 3126.66424274874 3050.66981206134 2975.60309908359 2901.43240753707 2828.12704567777 2755.6572786779 2683.9942834234 2613.11010557704 2542.97761876678 2473.57048576894 2404.8631215641 2336.83065815196 2269.44891101877;4143.00047553716 4049.21797528579 3956.76382674606 3865.59275021144 3775.66106220143 3686.92659703397 3599.34863271199 3512.88782084123 3427.50612031721 3343.16673453836 3259.83405191936 3177.4735894952 3096.05193942085 3015.5367181852 2935.89651837023 2857.10086279818 2779.12016091979 2701.92566730665 2625.48944211983 2549.78431343512;4598.50163279235 4494.40823886693 4391.78924195184 4290.59438407447 4190.77517898491 4092.28482510566 3995.07812326983 3899.11139893372 3804.34242857308 3710.73036999313 3618.23569630166 3526.82013331263 3436.44660016381 3347.079152947 3258.68293116342 3171.22410682959 3084.66983607064 2998.98821304921 2914.1482260877 2830.11971585147;5054.00279004754 4939.59850244808 4826.81465715762 4715.59601793749 4605.88929576838 4497.64305317735 4390.80761382767 4285.3349770262 4181.17873682896 4078.2940054479 3976.63734068395 3876.16667713006 3776.84126090677 3678.62158770879 3581.46934395661 3485.34735086099 ...(+2764 chars)]  NOMPRES=84000  PRESMAX=1000000  PRESMIN=10000  FNOMIN=750  FZMAX=8600  FZMIN=100  VXLOW=0.01  KPUMAX=AR26.KappaMax  KPUMIN=AR26.KappaMin  ALPMAX=1.5  ALPMIN=-1.5  CAMMAX=0.17453  CAMMIN=-0.17453  LONGVL=25  FxRelFreqLwrLim=200*pi  FyRelFreqLwrLim=200*pi  MyRelFreqLwrLim=100*pi  omegao=AR26.Omega0  UNLOADED_RADIUS=0.203  WIDTH=AR26.TireWidth  RIM_RADIUS=AR26.RimRadius  ASPECT_RATIO=0.45  MASS=11.2  IYY=1.084  br=1e-3  GRAVITY=-9.81  zo=0  zdoto=0  BREFF=8.25094594147963  DREFF=0.260468730454265  FREFF=0.0735298544471851  Q_RE0=1.00866439868088  Q_V1=0.000760413786224011  Q_V2=0.0463384792019201  Q_FZ1=0  Q_FZ2=15.6870832810226  Q_FZ3=0  Q_FCX=0.138643970247602  Q_FCY=0.10843499565426  Q_FCY2=-0.465763352339538  PFZ1=0.69958166705601  VERTICAL_STIFFNESS=207885.061134007  VERTICAL_DAMPING=500  BOTTOM_OFFST=0.00990653336182505  BOTTOM_STIFF=1999075.87051971  Q_CAM1=86.7791723017291  Q_CAM2=259.705254231766  Q_CAM3=0.510281667378416  Q_FYS1=-20769.4728880343  Q_FYS2=-59060.183485617  Q_FYS3=89271.8260126986  LONGITUDINAL_STIFFNESS=388714.175879854  LATERAL_STIFFNESS=157087.404633332  PCFX1=0.18539229191199  PCFX2=0  PCFX3=0  PCFY1=0.163183345037677  PCFY2=0  PCFY3=0.249094918231954  Q_RA1=0.675942571700787  Q_RA2=0.73800463546164  Q_RB1=1.04487486456705  Q_RB2=-1.191763806629  PCX1=1.5  PDX1=2.5435  PDX2=-0.64632  PDX3=11.0199  PEX1=-6.4596e-11  PEX2=-0.84982  PEX3=-0.6  PEX4=0.9  PKX1=42.6771  PKX2=-0.011985  PKX3=-0.53674  PHX1=0.0017597  PHX2=-0.001133  PVX1=-0.085025  PVX2=0.1  PPX1=0.25355  PPX2=12.2145  PPX3=-0.055934  PPX4=-2.6628  RBX1=5  RBX2=5  RBX3=0  RCX1=1  REX1=-1  REX2=-0.1  RHX1=0  QSX1=0  QSX2=1.5  QSX3=0.1  QSX4=0.1  QSX5=0  QSX6=0  QSX7=0.1  QSX8=0  QSX9=0  QSX10=0  QSX11=0  QSX12=0  QSX13=0  QSX14=0  PPMX1=0  PCY1=1.5  PDY1=2.1471  PDY2=-0.42791  PDY3=8.3327  PEY1=0.35224  PEY2=-0.17141  PEY3=0.10605  PEY4=-3.7833  PEY5=-62.9571  PKY1=-31.419  PKY2=1.5115  PKY3=0.30996  PKY4=2  PKY5=38.0826  PKY6=-3.9753  PKY7=-1.8011  PHY1=0.0024113  PHY2=0.00049845  PVY1=0.10412  PVY2=-0.053643  PVY3=0.53589  PVY4=1.2244  PPY1=0.40814  PPY2=1.0811  PPY3=-0.51005  PPY4=-0.29281  PPY5=-0.8874  RBY1=5  RBY2=2  RBY3=0.02  RBY4=0  RCY1=1  REY1=-0.1  REY2=0.1  RHY1=0  RHY2=0  RVY1=0  RVY2=0  RVY3=0  RVY4=0  RVY5=0  RVY6=0  QSY1=0  QSY2=0  QSY3=0  QSY4=0  QSY5=0  QSY6=0  QSY7=0  QSY8=0  QBZ1=0.36866  QBZ2=0.87296  QBZ3=0.64959  QBZ4=168.8149  QBZ5=-172.3075  QBZ6=0  QBZ9=-33.2482  QBZ10=-2.3968  QCZ1=14.2367  QDZ1=0.10605  QDZ2=-0.11593  QDZ3=4.9221  QDZ4=-8.2609  QDZ6=-0.023114  QDZ7=0.034508  QDZ8=-0.92786  QDZ9=2.4605  QDZ10=-11.696  QDZ11=-63.4068  QEZ1=-0.069508  QEZ2=-0.3322  QEZ3=-0.2814  QEZ4=3.6678  QEZ5=-275.1131  QHZ1=-0.019925  QHZ2=1.2787  QHZ3=-1.7534  QHZ4=0.77276  PPZ1=0  PPZ2=0  SSZ1=0  SSZ2=0  SSZ3=0  SSZ4=0  PDXP1=0  PDXP2=0  PDXP3=0  PKYP1=0  PDYP1=0  PDYP2=0  PDYP3=0  PDYP4=0  PHYP1=0  PHYP2=0  PHYP3=0  PHYP4=0  PECP1=0  PECP2=0  QDTP1=0  QCRP1=0  QCRP2=0  QBRP1=0  QDRP1=0  QDRP2=0  aMode=2
  Front Tyre Pressure : Constant  Value=AR26.FrontPressure
  Ground Displacement : Constant  Value=0
  ScaleFactors : Constant  Value=AR26.ScaleFctrs
  Out1 : Outport
  wires:
  Bus Creator/1 -> Out1/1
  Vx/1 -> Combined Slip Wheel 2DOF/3
  Front Tyre Pressure/1 -> Combined Slip Wheel 2DOF/7
  Ground Displacement/1 -> Combined Slip Wheel 2DOF/8
  Combined Slip Wheel 2DOF/2 -> Bus Creator/7  "omega"
  Combined Slip Wheel 2DOF/3 -> Bus Creator/8  "Fx"
  Vy/1 -> Combined Slip Wheel 2DOF/4
  Inclination Angle/1 -> Combined Slip Wheel 2DOF/5
  psidot/1 -> Combined Slip Wheel 2DOF/6
  Fz/1 -> Combined Slip Wheel 2DOF/9
  ScaleFactors/1 -> Combined Slip Wheel 2DOF/10
  Combined Slip Wheel 2DOF/5 -> Bus Creator/10
  Combined Slip Wheel 2DOF/6 -> Bus Creator/11
  Combined Slip Wheel 2DOF/7 -> Bus Creator/12
  Combined Slip Wheel 2DOF/8 -> Bus Creator/13
  BrkTrq/1 -> Combined Slip Wheel 2DOF/1
  DrvTrq/1 -> Combined Slip Wheel 2DOF/2  "axltrq"
  Combined Slip Wheel 2DOF/1 -> Bus Selector/1
  Bus Selector/5 -> Bus Creator/5  "<Vx>"
  Bus Selector/6 -> Bus Creator/6  "<Vy>"
  Bus Selector/1 -> Bus Creator/1  "<Alpha>"
  Bus Selector/2 -> Bus Creator/2  "<Kappa>"
  Bus Selector/3 -> Bus Creator/3  "<Gamma>"
  Bus Selector/4 -> Bus Creator/4  "<psidot>"
  Combined Slip Wheel 2DOF/4 -> Bus Creator/9  "Fy"
  Bus Selector/8 -> Bus Creator/15  "<WhlTrq>"
  Bus Selector/7 -> Bus Creator/14  "<AxlTrq>"

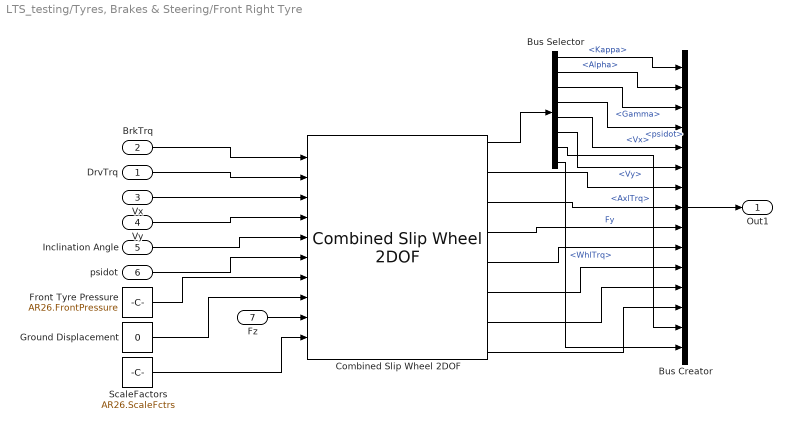
== system LTS_testing/Tyres, Brakes & Steering/Front Right Tyre ==
  DrvTrq : Inport
  BrkTrq : Inport  Port=2
  Vx : Inport  Port=3
  Vy : Inport  Port=4
  Inclination Angle : Inport  Port=5
  psidot : Inport  Port=6
  Fz : Inport  Port=7
  Bus Creator : BusCreator  Inputs=15
  Bus Selector : BusSelector  OutputSignals=Kappa,Alpha,Gamma,psidot,Vx,Vy,AxlTrq,WhlTrq
  Combined Slip Wheel 2DOF : vehdynlibtire/Combined Slip Wheel 2DOF  tireType=External file  tireParamSet=C:\Users\thoma\Documents\ME-Steering-2026\MATLAB\VD\right.tir  vertType=Magic Formula  plySteer=off  turnslip=off  BrakeType=Disc  mu_static=.3  mu_kinetic=.2  drum_abore=0.0508  drum_a=0.123  drum_c=0.212  drum_r=0.15  drum_theta1=0  drum_theta2=126  disk_abore=AR26.PistonDiam  Rm=AR26.DiscRadius  num_pads=AR26.NPistonAxle  brake_p_bpt=[1 11.4736842105263 21.9473684210526 32.4210526315789 42.8947368421053 53.3684210526316 63.8421052631579 74.3157894736842 84.7894736842105 95.2631578947368 105.736842105263 116.210526315789 126.684210526316 137.157894736842 147.631578947368 158.105263157895 168.578947368421 179.052631578947 189.526315789474 200]  brake_n_bpt=[0 52.6315789473684 105.263157894737 157.894736842105 210.526315789474 263.157894736842 315.789473684211 368.421052631579 421.052631578947 473.684210526316 526.315789473684 578.947368421053 631.578947368421 684.210526315789 736.842105263158 789.473684210526 842.105263157895 894.736842105263 947.368421052632 1000]  f_brake_t=[43.4900602404453 42.5056030554862 41.5350898940194 40.5780454442085 39.6340111501808 38.7025443887544 37.7832176914519 36.8756180088306 35.9793460143796 35.0940154454303 34.2192524787115 33.3546951383474 32.4999927342521 31.6548053290159 30.8188032315107 29.991666515561 29.1730845621415 28.362755623661 27.5603864089927 26.765691687993;498.991217495636 487.695866636631 476.560505099801 465.579679307235 454.748127933653 444.060772460445 433.51270824929 423.099196101319 412.81565427025 402.657650900201 392.620896861006 382.701238955775 372.894653477208 363.197240090814 353.605216024701 344.114910546964 334.722759712992 325.425301366216 316.219170376863 307.10109410434;954.492374750826 932.886130217776 911.585920305583 890.581313170261 869.862244717126 849.419000532136 829.242198807128 809.322774193808 789.651962526121 770.221286354971 751.0225412433 732.047782773203 713.289314220164 694.739674852612 676.391628817892 658.238154578366 640.272434863842 622.48784710877 604.877954344734 587.436496520688;1409.99353200602 1378.07639379892 1346.61133551136 1315.58294703329 1284.9763615006 1254.77722860383 1224.97168936497 1195.5463522863 1166.48827078199 1137.78492180974 1109.42418562559 1081.39432659063 1053.68397496312 1026.28210961441 999.178041611083 972.361398609768 945.822110014692 919.550392851325 893.536738312604 867.771898937035;1865.49468926121 1823.26665738007 1781.63675071715 1740.58458089631 1700.09047828407 1660.13545667552 1620.7011799228 1581.76993037878 1543.32457903786 1505.34855726451 1467.82583000789 1430.74087040806 1394.07863570608 1357.82454437621 1321.96445440427 1286.48464264117 1251.37178516554 1216.61293859388 1182.19552228048 1148.10730135338;2320.9958465164 2268.45692096121 2216.66216592293 2165.58621475934 2115.20459506754 2065.49368474721 2016.43067048064 1967.99350847127 1920.16088729373 1872.91219271928 1826.22747439018 1780.08741422549 1734.47329644903 1689.36697913801 1644.75086719747 1600.60788667257 1556.92146031639 1513.67548433643 1470.85430624835 1428.44270376973;2776.49700377159 2713.64718454235 2651.68758112871 2590.58784862237 2530.31871185102 2470.8519128189 2412.16016103848 2354.21708656376 2296.9971955496 2240.47582817405 2184.62911877248 2129.43395804292 2074.86795719199 2020.9094138998 1967.53727999066 1914.73113070398 1862.47113546724 1810.73803007899 1759.51309021622 1708.77810618608;3231.99816102678 3158.8374481235 3086.71299633449 3015.58948248539 2945.43282863449 2876.21014089059 2807.88965159632 2740.44066465625 2673.83350380547 2608.03946362882 2543.03076315477 2478.78050186034 2415.26261793494 2352.4518486616 2290.32369278385 2228.85437473538 2168.02081061809 2107.80057582154 2048.17187418409 1989.11350860242;3687.49931828197 3604.02771170464 3521.73841154027 3440.59111634842 3360.54694541796 3281.56836896228 3203.61914215416 3126.66424274874 3050.66981206134 2975.60309908359 2901.43240753707 2828.12704567777 2755.6572786779 2683.9942834234 2613.11010557704 2542.97761876678 2473.57048576894 2404.8631215641 2336.83065815196 2269.44891101877;4143.00047553716 4049.21797528579 3956.76382674606 3865.59275021144 3775.66106220143 3686.92659703397 3599.34863271199 3512.88782084123 3427.50612031721 3343.16673453836 3259.83405191936 3177.4735894952 3096.05193942085 3015.5367181852 2935.89651837023 2857.10086279818 2779.12016091979 2701.92566730665 2625.48944211983 2549.78431343512;4598.50163279235 4494.40823886693 4391.78924195184 4290.59438407447 4190.77517898491 4092.28482510566 3995.07812326983 3899.11139893372 3804.34242857308 3710.73036999313 3618.23569630166 3526.82013331263 3436.44660016381 3347.079152947 3258.68293116342 3171.22410682959 3084.66983607064 2998.98821304921 2914.1482260877 2830.11971585147;5054.00279004754 4939.59850244808 4826.81465715762 4715.59601793749 4605.88929576838 4497.64305317735 4390.80761382767 4285.3349770262 4181.17873682896 4078.2940054479 3976.63734068395 3876.16667713006 3776.84126090677 3678.62158770879 3581.46934395661 3485.34735086099 ...(+2764 chars)]  NOMPRES=84000  PRESMAX=1000000  PRESMIN=10000  FNOMIN=750  FZMAX=8600  FZMIN=100  VXLOW=0.01  KPUMAX=AR26.KappaMax  KPUMIN=AR26.KappaMin  ALPMAX=1.5  ALPMIN=-1.5  CAMMAX=0.17453  CAMMIN=-0.17453  LONGVL=25  FxRelFreqLwrLim=200*pi  FyRelFreqLwrLim=200*pi  MyRelFreqLwrLim=100*pi  omegao=AR26.Omega0  UNLOADED_RADIUS=0.203  WIDTH=AR26.TireWidth  RIM_RADIUS=AR26.RimRadius  ASPECT_RATIO=0.45  MASS=11.2  IYY=1.084  br=1e-3  GRAVITY=-9.81  zo=0  zdoto=0  BREFF=8.25094594147963  DREFF=0.260468730454265  FREFF=0.0735298544471851  Q_RE0=1.00866439868088  Q_V1=0.000760413786224011  Q_V2=0.0463384792019201  Q_FZ1=0  Q_FZ2=15.6870832810226  Q_FZ3=0  Q_FCX=0.138643970247602  Q_FCY=0.10843499565426  Q_FCY2=-0.465763352339538  PFZ1=0.69958166705601  VERTICAL_STIFFNESS=207885.061134007  VERTICAL_DAMPING=500  BOTTOM_OFFST=0.00990653336182505  BOTTOM_STIFF=1999075.87051971  Q_CAM1=86.7791723017291  Q_CAM2=259.705254231766  Q_CAM3=0.510281667378416  Q_FYS1=-20769.4728880343  Q_FYS2=-59060.183485617  Q_FYS3=89271.8260126986  LONGITUDINAL_STIFFNESS=388714.175879854  LATERAL_STIFFNESS=157087.404633332  PCFX1=0.18539229191199  PCFX2=0  PCFX3=0  PCFY1=0.163183345037677  PCFY2=0  PCFY3=0.249094918231954  Q_RA1=0.675942571700787  Q_RA2=0.73800463546164  Q_RB1=1.04487486456705  Q_RB2=-1.191763806629  PCX1=1.5  PDX1=2.5435  PDX2=-0.64632  PDX3=11.0199  PEX1=-6.4596e-11  PEX2=-0.84982  PEX3=-0.6  PEX4=0.9  PKX1=42.6771  PKX2=-0.011985  PKX3=-0.53674  PHX1=0.0017597  PHX2=-0.001133  PVX1=-0.085025  PVX2=0.1  PPX1=0.25355  PPX2=12.2145  PPX3=-0.055934  PPX4=-2.6628  RBX1=5  RBX2=5  RBX3=0  RCX1=1  REX1=-1  REX2=-0.1  RHX1=0  QSX1=0  QSX2=1.5  QSX3=0.1  QSX4=0.1  QSX5=0  QSX6=0  QSX7=0.1  QSX8=0  QSX9=0  QSX10=0  QSX11=0  QSX12=0  QSX13=0  QSX14=0  PPMX1=0  PCY1=1.5  PDY1=2.1471  PDY2=-0.42791  PDY3=8.3327  PEY1=0.35224  PEY2=-0.17141  PEY3=0.10605  PEY4=-3.7833  PEY5=-62.9571  PKY1=-31.419  PKY2=1.5115  PKY3=0.30996  PKY4=2  PKY5=38.0826  PKY6=-3.9753  PKY7=-1.8011  PHY1=0.0024113  PHY2=0.00049845  PVY1=0.10412  PVY2=-0.053643  PVY3=0.53589  PVY4=1.2244  PPY1=0.40814  PPY2=1.0811  PPY3=-0.51005  PPY4=-0.29281  PPY5=-0.8874  RBY1=5  RBY2=2  RBY3=0.02  RBY4=0  RCY1=1  REY1=-0.1  REY2=0.1  RHY1=0  RHY2=0  RVY1=0  RVY2=0  RVY3=0  RVY4=0  RVY5=0  RVY6=0  QSY1=0  QSY2=0  QSY3=0  QSY4=0  QSY5=0  QSY6=0  QSY7=0  QSY8=0  QBZ1=0.36866  QBZ2=0.87296  QBZ3=0.64959  QBZ4=168.8149  QBZ5=-172.3075  QBZ6=0  QBZ9=-33.2482  QBZ10=-2.3968  QCZ1=14.2367  QDZ1=0.10605  QDZ2=-0.11593  QDZ3=4.9221  QDZ4=-8.2609  QDZ6=-0.023114  QDZ7=0.034508  QDZ8=-0.92786  QDZ9=2.4605  QDZ10=-11.696  QDZ11=-63.4068  QEZ1=-0.069508  QEZ2=-0.3322  QEZ3=-0.2814  QEZ4=3.6678  QEZ5=-275.1131  QHZ1=-0.019925  QHZ2=1.2787  QHZ3=-1.7534  QHZ4=0.77276  PPZ1=0  PPZ2=0  SSZ1=0  SSZ2=0  SSZ3=0  SSZ4=0  PDXP1=0  PDXP2=0  PDXP3=0  PKYP1=0  PDYP1=0  PDYP2=0  PDYP3=0  PDYP4=0  PHYP1=0  PHYP2=0  PHYP3=0  PHYP4=0  PECP1=0  PECP2=0  QDTP1=0  QCRP1=0  QCRP2=0  QBRP1=0  QDRP1=0  QDRP2=0  aMode=2
  Front Tyre Pressure : Constant  Value=AR26.FrontPressure
  Ground Displacement : Constant  Value=0
  ScaleFactors : Constant  Value=AR26.ScaleFctrs
  Out1 : Outport
  wires:
  Front Tyre Pressure/1 -> Combined Slip Wheel 2DOF/7
  ScaleFactors/1 -> Combined Slip Wheel 2DOF/10
  psidot/1 -> Combined Slip Wheel 2DOF/6
  Vy/1 -> Combined Slip Wheel 2DOF/4
  Vx/1 -> Combined Slip Wheel 2DOF/3
  Ground Displacement/1 -> Combined Slip Wheel 2DOF/8
  Fz/1 -> Combined Slip Wheel 2DOF/9
  Inclination Angle/1 -> Combined Slip Wheel 2DOF/5
  DrvTrq/1 -> Combined Slip Wheel 2DOF/2
  BrkTrq/1 -> Combined Slip Wheel 2DOF/1
  Bus Creator/1 -> Out1/1
  Combined Slip Wheel 2DOF/2 -> Bus Creator/7
  Combined Slip Wheel 2DOF/8 -> Bus Creator/13
  Combined Slip Wheel 2DOF/7 -> Bus Creator/12
  Combined Slip Wheel 2DOF/6 -> Bus Creator/11
  Combined Slip Wheel 2DOF/5 -> Bus Creator/10
  Combined Slip Wheel 2DOF/3 -> Bus Creator/8
  Bus Selector/5 -> Bus Creator/5  "<Vx>"
  Bus Selector/6 -> Bus Creator/6  "<Vy>"
  Combined Slip Wheel 2DOF/1 -> Bus Selector/1
  Bus Selector/1 -> Bus Creator/1  "<Kappa>"
  Bus Selector/2 -> Bus Creator/2  "<Alpha>"
  Bus Selector/3 -> Bus Creator/3  "<Gamma>"
  Bus Selector/4 -> Bus Creator/4  "<psidot>"
  Combined Slip Wheel 2DOF/4 -> Bus Creator/9  "Fy"
  Bus Selector/8 -> Bus Creator/15  "<WhlTrq>"
  Bus Selector/7 -> Bus Creator/14  "<AxlTrq>"
